simulink model "freeHandGuiding_01"  (R2018a)
settings: Solver=FixedStepAuto  StartTime=0.0  StopTime=10000.0  RelTol=1e-3
undefined symbols (not defined in the file): DiscIntNeverNeededParam
libraries: dspnetwork x2, sldrtlib x1
settings Model: Creator=ronnie  LastModifiedBy=user

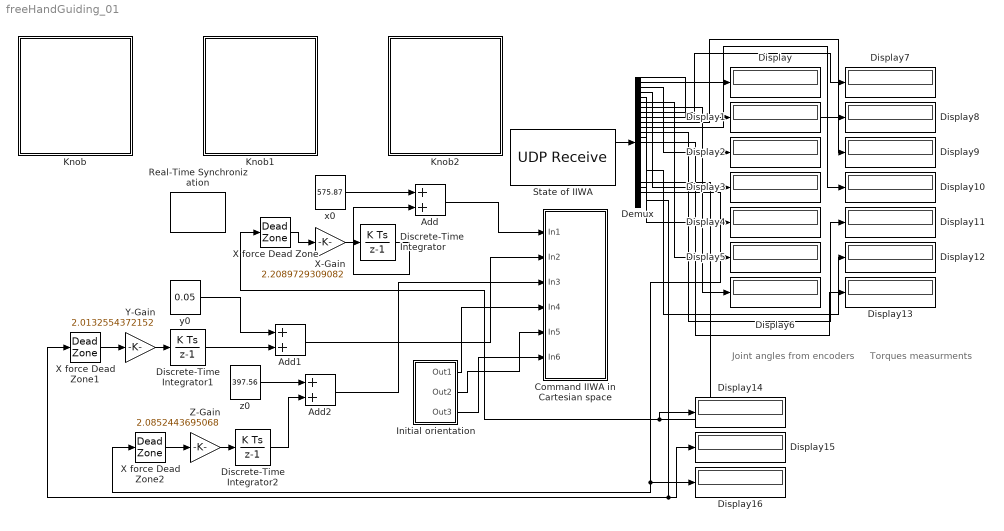
== system freeHandGuiding_01 ==
  note: Torques
      | measurments
  note: Joint angles from
      | encoders
  Add : Sum
  Add1 : Sum
  Add2 : Sum
  Command IIWA in Cartesian space : Subsystem
  Demux : Demux  Outputs=21+6
  Discrete-Time Integrator : DiscreteIntegrator  SampleTime=-1  ICPrevOutput=DiscIntNeverNeededParam  ICPrevScaledInput=DiscIntNeverNeededParam
  Discrete-Time Integrator1 : DiscreteIntegrator  SampleTime=-1  ICPrevOutput=DiscIntNeverNeededParam  ICPrevScaledInput=DiscIntNeverNeededParam
  Discrete-Time Integrator2 : DiscreteIntegrator  SampleTime=-1  ICPrevOutput=DiscIntNeverNeededParam  ICPrevScaledInput=DiscIntNeverNeededParam
  Display{,1..16} (17 alike) : Display
  "Initial orientation " : Subsystem
  Knob : Subsystem  DialogController=hmiCreateDDGDialog  IsWebBlock=on  mask(MWDashboardBlock){webBlockId=7b6023dd-8e9d-4e11-bff3-ec7cb6dff250, webBlockType=continuousknob, ShowInLibBrowser=on, ShowInitialText=on, HMISrcModelName=freeHandGuiding_01}
      mask prompts: webBlockId "WebBlock Id"; webBlockType "WebBlock Type"; HMISrcModelName "Source Model"
      mask help: SimulinkHMI:dialogs:ContinuousKnobDialogDesc
      mask Help: helpview([docroot '/mapfiles/simulink.map'], 'hmi_knob')
      mask Display:
      | if strcmp(get_param(bdroot(gcb),'BlockDiagramType'), 'library')
      |     image([(matlabroot) '/toolbox/simulink/hmi/icons/ContinuousKnob.png']);
      | end
  Knob1 : Subsystem  DialogController=hmiCreateDDGDialog  IsWebBlock=on  mask(MWDashboardBlock){webBlockId=86a47261-13e7-4ff7-8d8f-31be7ee4d310, webBlockType=continuousknob, ShowInLibBrowser=on, ShowInitialText=on, HMISrcModelName=freeHandGuiding_01}
      mask prompts: webBlockId "WebBlock Id"; webBlockType "WebBlock Type"; HMISrcModelName "Source Model"
      mask help: SimulinkHMI:dialogs:ContinuousKnobDialogDesc
      mask Help: helpview([docroot '/mapfiles/simulink.map'], 'hmi_knob')
      mask Display:
      | if strcmp(get_param(bdroot(gcb),'BlockDiagramType'), 'library')
      |     image([(matlabroot) '/toolbox/simulink/hmi/icons/ContinuousKnob.png']);
      | end
  Knob2 : Subsystem  DialogController=hmiCreateDDGDialog  IsWebBlock=on  mask(MWDashboardBlock){webBlockId=0b7cc13d-43d2-4f9f-a6d6-f0651e3aa515, webBlockType=continuousknob, ShowInLibBrowser=on, ShowInitialText=on, HMISrcModelName=freeHandGuiding_01}
      mask prompts: webBlockId "WebBlock Id"; webBlockType "WebBlock Type"; HMISrcModelName "Source Model"
      mask help: SimulinkHMI:dialogs:ContinuousKnobDialogDesc
      mask Help: helpview([docroot '/mapfiles/simulink.map'], 'hmi_knob')
      mask Display:
      | if strcmp(get_param(bdroot(gcb),'BlockDiagramType'), 'library')
      |     image([(matlabroot) '/toolbox/simulink/hmi/icons/ContinuousKnob.png']);
      | end
  Real-Time Synchronization : sldrtlib/Real-Time Synchronization  SampleTime=0.01  MaxMissedTicks=10  ShowMissedTicks=off  YieldWhenWaiting=off
  State of IIWA : dspnetwork/UDP Receive  localURL='0.0.0.0'  localPort=30008  remoteURL='172.31.1.147'  remotePort=-1  recvBufferSize=8192  dims=21+6  signalDatatype=double  isVarSize=off  showBlockingTime=off  blockingTime=0  sampletime=0.01  blockPlatform=[]
      settings: SourceProductName=DSP System Toolbox  SourceProductBaseCode=DS
  X force Dead Zone : DeadZone  LowerValue=-4  UpperValue=4  SaturateOnIntegerOverflow=on
  X force Dead Zone1 : DeadZone  LowerValue=-4  UpperValue=4  SaturateOnIntegerOverflow=on
  X force Dead Zone2 : DeadZone  LowerValue=-4  UpperValue=4  SaturateOnIntegerOverflow=on
  X-Gain : Gain  Gain=2.2089729309082
  Y-Gain : Gain  Gain=2.0132554372152
  Z-Gain : Gain  Gain=2.0852443695068
  x0 : Constant  Value=575.87  VectorParams1D=off  SampleTime=1/1000
  y0 : Constant  Value=0.05  VectorParams1D=off  SampleTime=1/1000
  z0 : Constant  Value=397.56  VectorParams1D=off  SampleTime=1/1000
  wires:
  Add2/1 -> Command IIWA in Cartesian space/3(In3)
  x0/1 -> Add/1
  Add/1 -> Command IIWA in Cartesian space/1(In1)
  Add1/1 -> Command IIWA in Cartesian space/2(In2)
  y0/1 -> Add1/1
  State of IIWA/1 -> Demux/1
  Demux/1 -> Display/1
  Demux/2 -> Display1/1
  Demux/3 -> Display2/1
  Demux/4 -> Display3/1
  Demux/5 -> Display4/1
  Demux/6 -> Display5/1
  Demux/7 -> Display6/1
  Demux/8 -> Display7/1
  Demux/9 -> Display8/1
  Demux/10 -> Display9/1
  Demux/11 -> Display10/1
  Demux/12 -> Display11/1
  Demux/13 -> Display12/1
  Demux/14 -> Display13/1
  Demux/24 -> X force Dead Zone2/1, Display16/1
  Demux/23 -> Display15/1, X force Dead Zone1/1
  Demux/22 -> Display14/1, X force Dead Zone/1
  X force Dead Zone/1 -> X-Gain/1
  X-Gain/1 -> Discrete-Time Integrator/1
  Discrete-Time Integrator/1 -> Add/2
  Discrete-Time Integrator1/1 -> Add1/2
  Y-Gain/1 -> Discrete-Time Integrator1/1
  X force Dead Zone1/1 -> Y-Gain/1
  "Initial orientation "/1(Out1) -> Command IIWA in Cartesian space/4(In4)
  "Initial orientation "/2(Out2) -> Command IIWA in Cartesian space/5(In5)
  "Initial orientation "/3(Out3) -> Command IIWA in Cartesian space/6(In6)
  z0/1 -> Add2/1
  X force Dead Zone2/1 -> Z-Gain/1
  Z-Gain/1 -> Discrete-Time Integrator2/1
  Discrete-Time Integrator2/1 -> Add2/2

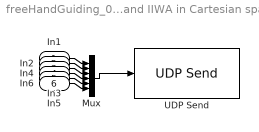
== system freeHandGuiding_01/Command IIWA in Cartesian space ==
  In1 : Inport
  In2 : Inport  Port=2
  In3 : Inport  Port=3
  In4 : Inport  Port=4
  In5 : Inport  Port=5
  In6 : Inport  Port=6
  Mux : Mux  Inputs=6
  UDP Send : dspnetwork/UDP Send  remoteURL='172.31.1.147'  remotePort=30002  localURL='0.0.0.0'  localPortSource=Automatically determine  localPort=-1  sampletime=-1  blockPlatform=[]  separateLengthPort=0
      settings: SourceProductName=DSP System Toolbox  SourceProductBaseCode=DS
  wires:
  Mux/1 -> UDP Send/1
  In3/1 -> Mux/3
  In5/1 -> Mux/5
  In2/1 -> Mux/2
  In1/1 -> Mux/1
  In6/1 -> Mux/6
  In4/1 -> Mux/4

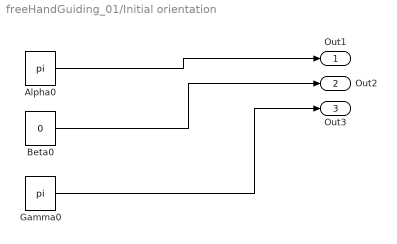
== system freeHandGuiding_01/Initial orientation  ==
  Alpha0 : Constant  Value=pi  VectorParams1D=off  SampleTime=1/1000
  Beta0 : Constant  Value=0  VectorParams1D=off  SampleTime=1/1000
  Gamma0 : Constant  Value=pi  VectorParams1D=off  SampleTime=1/1000
  Out1 : Outport
  Out2 : Outport  Port=2
  Out3 : Outport  Port=3
  wires:
  Alpha0/1 -> Out1/1
  Beta0/1 -> Out2/1
  Gamma0/1 -> Out3/1

== system freeHandGuiding_01/Knob ==

== system freeHandGuiding_01/Knob1 ==

== system freeHandGuiding_01/Knob2 ==
